simulink model "sampleModel1728"  (R2023a)
settings: Solver=VariableStepAuto  StartTime=0.0  StopTime=10.0  RelTol=1e-3
libraries: hdlsllib x3, simulink x3
settings Model: Creator=user1  LastModifiedBy=user1

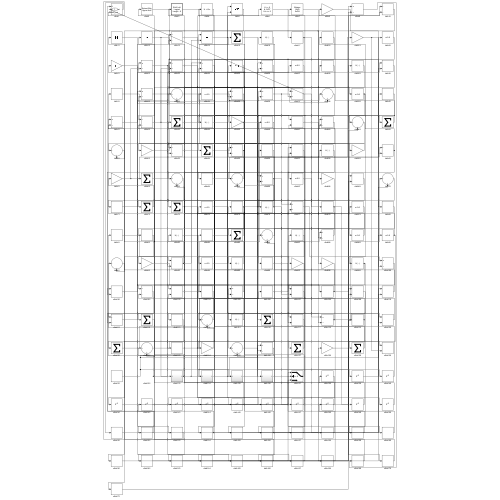
[thumbnail: Simulink's stored preview of the top-level diagram]
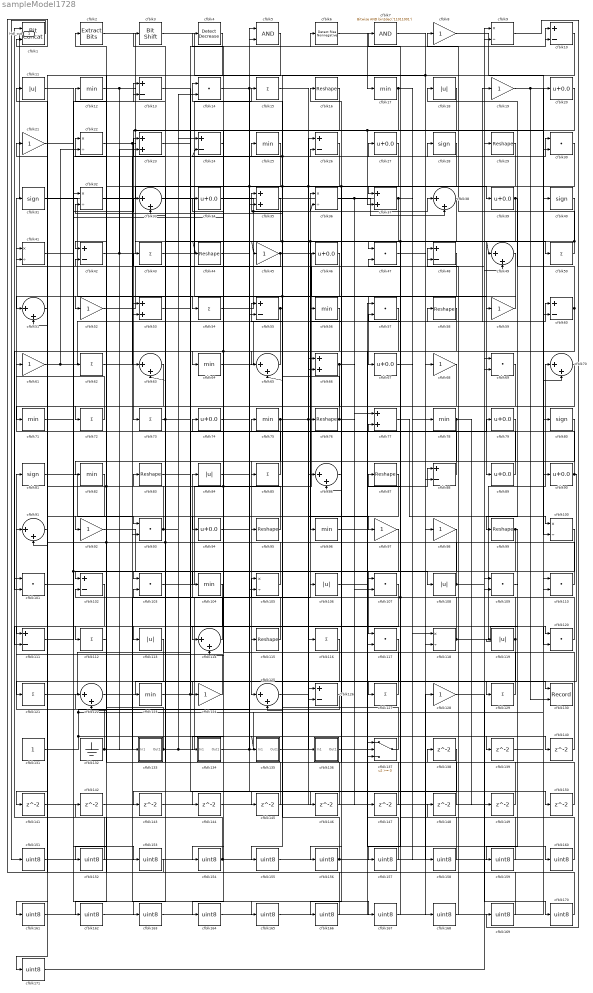
== system sampleModel1728 ==
  cfblk1 : hdlsllib/Logic and Bit Operations/Bit Concat  numInputs=2
  cfblk{10,13,24,26,42,48,55,60,88,102,111,126} (12 alike) : Sum  Inputs=+-  OutDataTypeStr=uint8
  cfblk{9,22,32,36,41,100,105,118} (8 alike) : Product  Inputs=*/  OutDataTypeStr=uint8  RndMeth=Zero  SaturateOnIntegerOverflow=on
  cfblk{14,30,47,57,69,93,101,103,107,109..110,117,120} (13 alike) : DotProduct  OutDataTypeStr=uint8
  cfblk{12,17,25,56,64,71,75,78,82,96,104,123} (12 alike) : MinMax  OutDataTypeStr=uint8
  cfblk{11,18,84,106,108,113,119} (7 alike) : Abs  OutDataTypeStr=uint8  SaturateOnIntegerOverflow=off
  cfblk{15,43,50,54,62,72..73,85,112,116,121,127,129} (13 alike) : Sum  Inputs=+  OutDataTypeStr=uint8
  cfblk{33,38,49,51,63,65,70,86,91,114,122,125} (12 alike) : Sum  Inputs=|++  OutDataTypeStr=uint8
  cfblk{16,29,44,58,76,83,87,95,99,115} (10 alike) : Reshape
  cfblk{8,19,21,45,52,59,61,68,92,97..98,124,128} (13 alike) : Gain  OutDataTypeStr=uint8
  cfblk130 : Record  FileSettingsInternal="{\"entries\":[{\"content\":{\"excelSettings\":{\"content\":{},\"type\":\"Streamout.ExcelSettings\"}},\"type\":\"Streamout.FileSettingStorage\",\"uuid\":\"\"}],\"packageUris\":[\"http:\\/\\/schema.mathworks.com\\/mf0\\/streamout_blocks\\/R2020a\"],\"version\":\"1.0\"}"  Layout=[1 1]  SignalsInternal="{\"entries\":[{\"content\":{\"signals\":[{\"content\":{\"blockPath\":[],\"dimensions\":[1],\"domain\":\"\",\"lineColor\":\"#a2142f\",\"plots\":[1],\"port\":1,\"signalID\":38078,\"signalName\":\"cfblk122\"},\"type\":\"RecordBlkView.Signal\",\"uuid\":\"\"},{\"content\":{\"blockPath\":[],\"dimensions\":[1],\"domain\":\"\",\"lineColor\":\"#139fff\",\"plots\":[1],\"port\":2,\"signalID\":38081,\"signalName\":\"cfblk19\"},\"type\":\"RecordBlkView.Signal\",\"uuid\":\"\"}]},\"type\":\"RecordBlkView.InputSignals\",\"uuid\":\"\"}],\"packageUris\":[\"http:\\/\\/schema.mathworks.com\\/mf0\\/streamout_blocks\\/R2020a\"],\"version\":\"1.0\"}"  VisualizationBindings="{\"xyplotplugin\":{\"info\":[{\"series\":[{\"bindingParametersList\":[{\"parameter\":\"X-Axis\",\"signalID\":38078,\"signalName\":\"cfblk122\"},{\"parameter\":\"Y-Axis\",\"signalID\":38081,\"signalName\":\"cfblk19\"}],\"seriesID\":20376}],\"subplotID\":1}]}}"  CompatibilityTag=XY  st=-1
  cfblk131 : Constant  OutDataTypeStr=uint8  SampleTime=-1
  cfblk132 : Ground
  cfblk133 : Subsystem
      settings: LibrarySourceBlock=|
      | hdlsllib/Ports &
      | Subsystems/Subsystem
  cfblk134 : Subsystem
      settings: LibrarySourceBlock=|
      | hdlsllib/Ports &
      | Subsystems/Subsystem
  cfblk135 : Subsystem
      settings: LibrarySourceBlock=|
      | hdlsllib/Ports &
      | Subsystems/Subsystem
  cfblk136 : Subsystem
      settings: LibrarySourceBlock=|
      | hdlsllib/Ports &
      | Subsystems/Subsystem
  cfblk137 : Switch  OutDataTypeStr=uint8  SaturateOnIntegerOverflow=off  InputSameDT=off
  cfblk{138..150} (13 alike) : Delay  SampleTime=1
  cfblk{151..171} (21 alike) : DataTypeConversion  OutDataTypeStr=uint8  SaturateOnIntegerOverflow=off  RndMeth=Floor
  cfblk2 : simulink/Logic and Bit Operations/Extract Bits  bitsToExtract=Upper half  numBits=8  bitIdxRange=[0 7]  outScalingMode=Preserve fixed-point scaling
      settings: LibrarySourceBlock=|
      | hdlsllib/Logic and Bit
      | Operations/Extract Bits
  cfblk{20,27,34,39,46,67,74,79,89..90,94} (11 alike) : Bias  Bias=0.0  SaturateOnIntegerOverflow=off
  cfblk{23,35,37,53,66,77} (6 alike) : Sum  OutDataTypeStr=uint8
  cfblk{28,31,40,80..81} (5 alike) : Signum
  cfblk3 : hdlsllib/Logic and Bit Operations/Bit Shift  mode=Shift Left Logical  N=0
  cfblk4 : simulink/Logic and Bit Operations/Detect Decrease  vinit=0.0  OutDataTypeStr=uint8
      settings: LibrarySourceBlock=|
      | hdlsllib/Logic and Bit
      | Operations/Detect
      | Decrease
  cfblk5 : Logic  AllPortsSameDT=off  OutDataTypeStr=boolean
  cfblk6 : hdlsllib/Logic and Bit Operations/Detect Rise Nonnegative  vinit=0  OutDataTypeStr=uint8
  cfblk7 : simulink/Logic and Bit Operations/Bitwise Operator  logicop=AND  UseBitMask=on  BitMask=bin2dec('11011001')  BitMaskRealWorld=Stored Integer
      settings: LibrarySourceBlock=|
      | hdlsllib/Logic and Bit
      | Operations/Bitwise
      | Operator
  Hdl_out : Outport  OutDataTypeStr=uint8
  wires:
  cfblk16/1 -> cfblk73/1
  cfblk57/1 -> cfblk156/1
  cfblk31/1 -> cfblk54/1
  cfblk67/1 -> cfblk78/1
  cfblk39/1 -> cfblk89/1, cfblk99/1
  cfblk55/1 -> cfblk113/1, cfblk35/1
  cfblk72/1 -> cfblk31/1
  cfblk77/1 -> cfblk100/1
  cfblk114/1 -> cfblk84/1
  cfblk75/1 -> cfblk19/1, cfblk27/1, cfblk134/1(In1)
  cfblk78/1 -> cfblk149/1, cfblk166/1
  cfblk65/1 -> cfblk63/1
  cfblk93/1 -> cfblk83/1, cfblk24/1
  cfblk90/1 -> cfblk129/1, cfblk13/2
  cfblk126/1 -> cfblk81/1
  cfblk103/1 -> cfblk48/1
  cfblk70/1 -> cfblk72/1
  cfblk22/1 -> cfblk66/1, cfblk167/1
  cfblk79/1 -> cfblk125/1
  cfblk6/1 -> cfblk17/1
  cfblk18/1 -> cfblk104/1
  cfblk122/1 -> cfblk130/1
  cfblk47/1 -> cfblk98/1
  cfblk123/1 -> cfblk36/1, cfblk10/1
  cfblk88/1 -> cfblk61/1
  cfblk37/1 -> cfblk96/1, cfblk44/1, cfblk118/1, Hdl_out/1
  cfblk124/1 -> cfblk91/1
  cfblk133/1(Out1) -> cfblk5/1, cfblk14/2, cfblk22/1
  cfblk42/1 -> cfblk50/1, cfblk23/2
  cfblk118/1 -> cfblk70/1, cfblk105/1
  cfblk137/1 -> cfblk32/2
  cfblk17/1 -> cfblk37/2, cfblk155/1, cfblk158/1
  cfblk63/1 -> cfblk91/2
  cfblk98/1 -> cfblk102/1
  cfblk99/1 -> cfblk119/1, cfblk157/1
  cfblk86/1 -> cfblk16/1
  cfblk50/1 -> cfblk49/1, cfblk8/1
  cfblk54/1 -> cfblk59/1
  cfblk100/1 -> cfblk112/1
  cfblk92/1 -> cfblk108/1
  cfblk76/1 -> cfblk14/1, cfblk24/2, cfblk107/2
  cfblk110/1 -> cfblk56/1
  cfblk104/1 -> cfblk114/1
  cfblk85/1 -> cfblk75/1
  cfblk97/1 -> cfblk117/1
  cfblk45/1 -> cfblk67/1, cfblk41/2
  cfblk32/1 -> cfblk37/1
  cfblk33/1 -> cfblk136/1(In1)
  cfblk108/1 -> cfblk74/1, cfblk10/2
  cfblk129/1 -> cfblk87/1
  cfblk11/1 -> cfblk105/2, cfblk153/1
  cfblk127/1 -> cfblk43/1
  cfblk73/1 -> cfblk103/1, cfblk77/2
  cfblk38/1 -> cfblk107/1, cfblk53/1
  cfblk83/1 -> cfblk120/1
  cfblk29/1 -> cfblk114/2, cfblk35/2
  cfblk116/1 -> cfblk126/2
  cfblk120/1 -> cfblk55/1
  cfblk12/1 -> cfblk39/1, cfblk60/2, cfblk133/1(In1)
  cfblk131/1 -> cfblk5/2, cfblk30/2, cfblk135/1(In1)
  cfblk87/1 -> cfblk92/1
  cfblk115/1 -> cfblk102/2
  cfblk121/1 -> cfblk79/1
  cfblk8/1 -> cfblk80/1
  cfblk44/1 -> cfblk55/2
  cfblk82/1 -> cfblk111/1
  cfblk48/1 -> cfblk95/1
  cfblk25/1 -> cfblk93/1
  cfblk59/1 -> cfblk51/1
  cfblk27/1 -> cfblk64/1
  cfblk43/1 -> cfblk15/1
  cfblk94/1 -> cfblk46/1
  cfblk40/1 -> cfblk94/1
  cfblk135/1(Out1) -> cfblk38/1
  cfblk64/1 -> cfblk40/1
  cfblk19/1 -> cfblk100/2, cfblk130/2
  cfblk36/1 -> cfblk38/2, cfblk147/1
  cfblk2/1 -> cfblk47/1
  cfblk51/1 -> cfblk71/1
  cfblk81/1 -> cfblk123/1
  cfblk34/1 -> cfblk116/1, cfblk36/2
  cfblk49/1 -> cfblk93/2
  cfblk119/1 -> cfblk47/2, cfblk34/1, cfblk127/1
  cfblk15/1 -> cfblk97/1
  cfblk106/1 -> cfblk88/1
  cfblk5/1 -> cfblk51/2
  cfblk89/1 -> cfblk23/1
  cfblk58/1 -> cfblk117/2
  cfblk60/1 -> cfblk125/2, cfblk18/1
  cfblk68/1 -> cfblk85/1
  cfblk28/1 -> cfblk76/1, cfblk53/2
  cfblk14/1 -> cfblk6/1, cfblk118/2
  cfblk35/1 -> cfblk124/1
  cfblk62/1 -> cfblk30/1
  cfblk4/1 -> cfblk42/1
  cfblk41/1 -> cfblk33/1
  cfblk105/1 -> cfblk2/1, cfblk41/1, cfblk63/2
  cfblk3/1 -> cfblk68/1
  cfblk132/1 -> cfblk122/1, cfblk106/1
  cfblk107/1 -> cfblk111/2
  cfblk84/1 -> cfblk120/2
  cfblk66/1 -> cfblk77/1, cfblk143/1
  cfblk91/1 -> cfblk121/1
  cfblk46/1 -> cfblk115/1, cfblk82/1
  cfblk71/1 -> cfblk13/1
  cfblk134/1(Out1) -> cfblk86/1, cfblk28/1
  cfblk95/1 -> cfblk11/1, cfblk12/1, cfblk4/1
  cfblk112/1 -> cfblk122/2
  cfblk101/1 -> cfblk26/2
  cfblk52/1 -> cfblk29/1
  cfblk61/1 -> cfblk60/1, cfblk22/2
  cfblk30/1 -> cfblk65/1, cfblk33/2
  cfblk56/1 -> cfblk101/2, cfblk164/1
  cfblk26/1 -> cfblk52/1, cfblk66/2
  cfblk111/1 -> cfblk62/1
  cfblk10/1 -> cfblk45/1, cfblk65/2, cfblk88/2
  cfblk136/1(Out1) -> cfblk58/1
  cfblk20/1 -> cfblk154/1
  cfblk13/1 -> cfblk139/1
  cfblk139/1 -> cfblk70/2
  cfblk125/1 -> cfblk140/1
  cfblk140/1 -> cfblk32/1
  cfblk117/1 -> cfblk141/1
  cfblk141/1 -> cfblk137/2
  cfblk142/1 -> cfblk137/1
  cfblk143/1 -> cfblk26/1
  cfblk24/1 -> cfblk144/1
  cfblk144/1 -> cfblk49/2
  cfblk23/1 -> cfblk145/1
  cfblk145/1 -> cfblk42/2
  cfblk53/1 -> cfblk146/1
  cfblk146/1 -> cfblk103/2
  cfblk147/1 -> cfblk3/1
  cfblk148/1 -> cfblk126/1
  cfblk149/1 -> cfblk86/2
  cfblk74/1 -> cfblk150/1
  cfblk150/1 -> cfblk48/2
  cfblk1/1 -> cfblk151/1
  cfblk151/1 -> cfblk110/2
  cfblk80/1 -> cfblk152/1
  cfblk152/1 -> cfblk1/1
  cfblk153/1 -> cfblk1/2
  cfblk154/1 -> cfblk90/1, cfblk101/1
  cfblk155/1 -> cfblk20/1
  cfblk156/1 -> cfblk128/1, cfblk25/1
  cfblk157/1 -> cfblk57/1
  cfblk158/1 -> cfblk57/2
  cfblk109/1 -> cfblk159/1
  cfblk159/1 -> cfblk138/1
  cfblk96/1 -> cfblk160/1
  cfblk160/1 -> cfblk109/1
  cfblk102/1 -> cfblk161/1
  cfblk161/1 -> cfblk109/2
  cfblk69/1 -> cfblk162/1
  cfblk162/1 -> cfblk137/3
  cfblk138/1 -> cfblk163/1
  cfblk163/1 -> cfblk69/1
  cfblk164/1 -> cfblk69/2
  cfblk21/1 -> cfblk165/1
  cfblk165/1 -> cfblk110/1
  cfblk166/1 -> cfblk21/1
  cfblk167/1 -> cfblk7/1
  cfblk7/1 -> cfblk168/1
  cfblk168/1 -> cfblk148/1
  cfblk9/1 -> cfblk169/1
  cfblk169/1 -> cfblk142/1
  cfblk128/1 -> cfblk170/1
  cfblk170/1 -> cfblk9/1
  cfblk113/1 -> cfblk171/1
  cfblk171/1 -> cfblk9/2

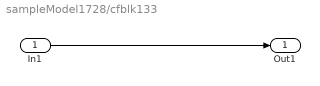
== system sampleModel1728/cfblk133 ==
  In1 : Inport
  Out1 : Outport
  wires:
  In1/1 -> Out1/1

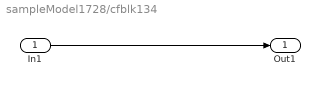
== system sampleModel1728/cfblk134 ==
  In1 : Inport
  Out1 : Outport
  wires:
  In1/1 -> Out1/1

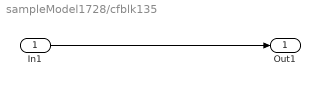
== system sampleModel1728/cfblk135 ==
  In1 : Inport
  Out1 : Outport
  wires:
  In1/1 -> Out1/1

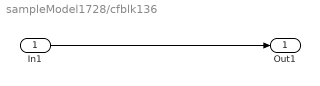
== system sampleModel1728/cfblk136 ==
  In1 : Inport
  Out1 : Outport
  wires:
  In1/1 -> Out1/1
